simulink model "fft_4096c_1i_core"  (R2019a)
(part 5 of 150)

  butterfly3_7 : Subsystem  AncestorBlock=casper_library_ffts/butterfly_direct  mask(butterfly_direct){n_inputs=1, biplex=off, FFTSize=13, Coeffs=[ 7 2055 1031 3079 519 2567 1543 3591 263 2311 1287 3335 775 2823 1799 3847 135 2183 1159 3207 647 2695 1671 3719 391 2439 1415 3463 903 2951 1927 3975 71 2119 1095 3143 583 2631 1607 3655 327 2375 1351 3399 839 2887 1863 3911 199 2247 1223 3271 711 2759 1735 3783 455 2503 1479 3527 967 3015 1991 4039 39 2087 1063 3111 551 2599 1575 3623 295 2343 1319 3367 807 2855 1831 3879 167 2215 1191 3239 679 2727 1703 3751 423 2471 1447 3495 935 2983 1959 4007 103 2151 1127 3175 615 2663 1639 3687 359 2407 1383 3431 871 2919 1895 3943 231 2279 1255 3303 743 2791 1767 3815 487 2535 1511 3559 999 3047 2023 4071 23 2071 1047 3095 535 2583 1559 3607 279 2327 1303 3351 791 2839 1815 3863 151 2199 1175 3223 663 2711 1687 3735 407 2455 1431 3479 919 2967 1943 3991 87 2135 1111 3159 599 2647 1623 3671 343 2391 1367 3415 855 2903 1879 3927 215 2263 1239 3287 727 2775 1751 3799 471 2519 1495 3543 983 3031 2007 4055 55 2103 1079 3127 567 2615 1591 3639 311 2359 1335 3383 823 2871 1847 3895 183 2231 1207 3255 695 2743 1719 3767 439 2487 1463 3511 951 2999 1975 4023 119 2167 1143 3191 631 2679 1655 3703 375 2423 1399 3447 887 2935 1911 3959 247 2295 1271 3319 759 2807 1783 3831 503 2551 1527 3575 1015 3063 2039 4087 15 2063 1039 3087 527 2575 1551 3599 271 2319 1295 3343 783 2831 1807 3855 143 2191 1167 3215 655 2703 1679 3727 399 2447 1423 3471 911 2959 1935 3983 79 2127 1103 3151 591 2639 1615 3663 335 2383 1359 3407 847 2895 1871 3919 207 2255 1231 3279 719 2767 1743 3791 463 2511 1487 3535 975 3023 1999 4047 47 2095 1071 3119 559 2607 1583 3631 303 2351 1327 3375 815 2863 1839 3887 175 2223 1199 3247 687 2735 1711 3759 431 2479 1455 3503 943 2991 1967 4015 111 2159 1135 3183 623 2671 1647 3695 367 2415 1391 3439 879 2927 1903 3951 239 2287 1263 3311 751 2799 1775 3823 495 2543 1519 3567 1007 3055 2031 4079 31 2079 1055 3103 543 2591 1567 3615 287 2335 1311 3359 799 2847 1823 3871 159 2207 1183 3231 671 2719 1695 3743 415 2463 1439 3487 927 2975 1951 3999 95 2143 1119 3167 607 2655 1631 3679 351 2399 1375 3423 863 2911 1887 3935 223 2271 1247 3295 735 2783 1759 3807 479 2527 1503 3551 991 3039 2015 4063 63 2111 1087 3135 575 2623 1599 3647 319 2367 1343 3391 831 2879 1855 3903 191 2239 1215 3263 703 2751 1727 3775 447 2495 1471 3519 959 3007 1983 4031 127 2175 1151 3199 639 2687 1663 3711 383 2431 1407 3455 895 2943 1919 3967 255 2303 1279 3327 767 2815 1791 3839 511 2559 1535 3583 1023 3071 2047 4095], StepPeriod=0, coeff_bit_width=18, input_bit_width=18, bin_pt_in=17, downshift=off, async=off, floating_point=off, float_type=single, exp_width=8, frac_width=24, add_latency=1, mult_latency=2, bram_latency=2, conv_latency=0, add_pipe_latency=0, mult_pipe_latency=0, quantization=Round  (unbiased: Even Values), overflow=Wrap, coeffs_bit_limit=8, coeff_sharing=on, coeff_decimation=on, coeff_generation=off, cal_bits=1, n_bits_rotation=25, max_fanout=8, use_hdl=on, use_embedded=off, bitgrowth=off, hardcode_shifts=off, dsp48_adders=off}
      mask prompts: n_inputs "number inputs"; biplex "Used in biplex FFT"; FFTSize "Size of FFT: (2^? pts)"; Coeffs "Coefficients: (0 to 2^(FFTSize-1)-1)"; StepPeriod "Coefficient Step Period: (2^?)"; coeff_bit_width "Coefficient Bit Width"; input_bit_width "Input Bit Width"; bin_pt_in "Input binary point"; async "asynchronous operation"; floating_point "floating point"; float_type "float type"; exp_width "exponent width"; frac_width "fraction width"; add_latency "Add Latency"; mult_latency "Mult Latency"; bram_latency "BRAM Latency"; conv_latency "Convert latency"; add_pipe_latency "Add Pipeline Latency"; mult_pipe_latency "Mult Pipeline Latency"; quantization "Quantization Behavior"; overflow "Overflow Behavior"; coeffs_bit_limit "Number bits above which to store stage's coefficients in BRAM (2^? bits)"; coeff_sharing "BRAM sharing in coeff storage"; coeff_decimation "Store a fraction of coeff factors where useful"; coeff_generation "Generate coeffs with multipliers where useful"; cal_bits "Number calibration locations when generating coeffs (2^?)"; n_bits_rotation "Feedback rotation vector resolution"; max_fanout "Maximum fanout"; use_hdl "Use behavioural HDL for multipliers"; use_embedded "Use embedded multipliers"; bitgrowth "Bit growth instead of shifting"; hardcode_shifts "Hardcode shift schedule"; dsp48_adders "Use DSP48s for adders"
      mask help: FFT internal block.
      mask init: same as fft_4096c_1i_core/fft_wideband_real1/fft_direct/butterfly0_0
      settings: AttributesFormatString=twiddle_general
      mask Callback floating_point:
      | onoff = get_param(gcb, 'floating_point');
      | if strcmp(onoff,'on')
      |     enable_fixpt = 'off';
      |     set_param_state(gcb, 'float_type', 'on')
      | 
      |     f_type = get_param(gcb, 'float_type');
      |     if strcmp(f_type,'custom')
      |         set_param_state(gcb, 'exp_width', 'on')
      |         set_param_state(gcb, 'frac_width', 'on')
      |     else
      |         set_param_state(gcb, 'exp_width', 'off')
      |         set_param_state(gcb, 'frac_width', 'off')
      |     end
      | 
      | 
      | else
      |     enable_fixpt = 'on';
      |     set_param_state(gcb, 'float_type', 'off')
      |     set_param_state(gcb, 'exp_width', 'off')
      |     set_param_state(gcb, 'frac_width', 'off')
      | end
      | 
      | set_param_state(gcb, 'input_bit_width', enable_fixpt)
      | set_param_state(gcb, 'bin_pt_in', enable_fixpt)
      | set_param_state(gcb, 'coeff_bit_width', enable_fixpt)
      mask TypeOptions float_type: single | custom
      mask Callback float_type:
      | f_type = get_param(gcb, 'float_type')
      | if strcmp(f_type,'custom')
      |     set_param_state(gcb, 'exp_width', 'on')
      |     set_param_state(gcb, 'frac_width', 'on')
      | else
      |     set_param_state(gcb, 'exp_width', 'off')
      |     set_param_state(gcb, 'frac_width', 'off')
      | end
      mask TypeOptions quantization: Truncate | Round  (unbiased: +/- Inf) | Round  (unbiased: Even Values)
      mask TypeOptions overflow: Wrap | Saturate | Error
      mask Callback use_hdl:
      | % make mutually exclusive with use_embedded.
      | 
      | use_hdl = get_param(gcb, 'use_hdl');
      | if strcmp(use_hdl, 'on'),
      |     set_param_state(gcb, 'use_embedded', 'off');
      | else
      |     set_param_state(gcb, 'use_embedded', 'on');
      | end
      mask Callback use_embedded:
      | % make mutually exclusive with use_hdl.
      | 
      | use_hdl = get_param(gcb, 'use_embedded');
      | if strcmp(use_hdl, 'on'),
      |     set_param_state(gcb, 'use_hdl', 'off');
      | else
      |     set_param_state(gcb, 'use_hdl', 'on');
      | end
      mask Callback hardcode_shifts:
      | hardcode_shifts = get_param(gcb, 'hardcode_shifts');
      | set_param_state(gcb, 'downshift', hardcode_shifts);
      mask Callback dsp48_adders: %fft_callback_dsp48_adders(gcb);
      mask DialogControl ParameterTabVar0 Prompt: Basic
      mask DialogControl ParameterTabVar01 Prompt: Latency
      mask DialogControl ParameterTabVar012 Prompt: Implementation
  combine : xbsIndex_r4/Logical  logical_function=OR  inputs=8  en=off  latency=2  precision=Full  arith_type=Unsigned  n_bits=16  bin_pt=0  align_bp=on  dbl_ovrd=off  block_type=logical
  of_0 : xbsIndex_r4/Delay  rst=off  infoeditControl=Selection of Reset will increase slice count due to use of real FFs and instead of SRLs  en=off  latency=0  reg_retiming=on  dbl_ovrd=off  block_type=delay
  of_1 : xbsIndex_r4/Concat  num_inputs=2  dbl_ovrd=off  block_type=concat
  of_2 : xbsIndex_r4/Concat  num_inputs=4  dbl_ovrd=off  block_type=concat
  of_3 : xbsIndex_r4/Concat  num_inputs=8  dbl_ovrd=off  block_type=concat
  of_expand : Subsystem  AncestorBlock=casper_library_flow_control/bus_expand  mask(bus_expand){mode=divisions of equal size, outputNum=8, outputWidth=1, outputBinaryPt=0, outputArithmeticType=0, show_format=off, outputToWorkspace=off, variablePrefix=out, outputToModelAsWell=on}
      mask prompts: outputNum "Number of outputs:"; outputWidth "Output width:"; outputBinaryPt "Output binary point position:"; outputArithmeticType "Output arithmetic type (ufix=0, fix=1, bool=2):"; show_format "Print format string?"; outputToWorkspace "Output to workspace?"; variablePrefix "Variable name prefix:"; outputToModelAsWell "Output to model as well?"
      mask help:
      | Expands a 'bus' made using a bus_create or Xilinx
      | concat block.
      | The input will be divided into the specified number
      | of outputs with the specified arithmetic types.
      | Divisions are made from most significant bit.
      mask init: same as fft_4096c_1i_core/bus_expand
      settings: AttributesFormatString=8 outputs
      mask TypeOptions mode: divisions of equal size | divisions of arbitrary size
      mask Callback mode: bus_expand_callback();
      mask Callback outputWidth: bus_expand_callback();
      mask Callback outputToWorkspace: bus_expand_callback();
  of_or : xbsIndex_r4/Logical  logical_function=OR  inputs=4  en=off  latency=2  precision=Full  arith_type=Unsigned  n_bits=16  bin_pt=0  align_bp=on  dbl_ovrd=off  block_type=logical
  slice0 : xbsIndex_r4/Slice  nbits=1  boolean_output=on  mode=Lower Bit Location + Width  bit1=0  base1=MSB of Input  bit0=0  base0=LSB of Input  dbl_ovrd=off  block_type=slice
  slice1 : xbsIndex_r4/Slice  nbits=1  boolean_output=on  mode=Lower Bit Location + Width  bit1=0  base1=MSB of Input  bit0=1  base0=LSB of Input  dbl_ovrd=off  block_type=slice
  slice2 : xbsIndex_r4/Slice  nbits=1  boolean_output=on  mode=Lower Bit Location + Width  bit1=0  base1=MSB of Input  bit0=2  base0=LSB of Input  dbl_ovrd=off  block_type=slice
  slice3 : xbsIndex_r4/Slice  nbits=1  boolean_output=on  mode=Lower Bit Location + Width  bit1=0  base1=MSB of Input  bit0=3  base0=LSB of Input  dbl_ovrd=off  block_type=slice
  synct{1..7} (7 alike) : Terminator
  sync_out : Outport
  out00 : Outport  Port=2
  out01 : Outport  Port=3
  out02 : Outport  Port=4
  out03 : Outport  Port=5
  out04 : Outport  Port=6
  out05 : Outport  Port=7
  out06 : Outport  Port=8
  out07 : Outport  Port=9
  out08 : Outport  Port=10
  out09 : Outport  Port=11
  out010 : Outport  Port=12
  out011 : Outport  Port=13
  out012 : Outport  Port=14
  out013 : Outport  Port=15
  out014 : Outport  Port=16
  out015 : Outport  Port=17
  of : Outport  Port=18
  wires:
  in00/1 -> abus/1(in1)
  adebus3_0/1(msb_lsb_out1) -> out00/1
  in01/1 -> abus/2(in2)
  adebus3_4/1(msb_lsb_out1) -> out01/1
  in02/1 -> abus/3(in3)
  adebus3_2/1(msb_lsb_out1) -> out02/1
  in03/1 -> abus/4(in4)
  adebus3_6/1(msb_lsb_out1) -> out03/1
  in04/1 -> abus/5(in5)
  adebus3_1/1(msb_lsb_out1) -> out04/1
  in05/1 -> abus/6(in6)
  adebus3_5/1(msb_lsb_out1) -> out05/1
  in06/1 -> abus/7(in7)
  adebus3_3/1(msb_lsb_out1) -> out06/1
  in07/1 -> abus/8(in8)
  adebus3_7/1(msb_lsb_out1) -> out07/1
  in08/1 -> bbus/1(in1)
  bdebus3_0/1(msb_lsb_out1) -> out08/1
  in09/1 -> bbus/2(in2)
  bdebus3_4/1(msb_lsb_out1) -> out09/1
  in010/1 -> bbus/3(in3)
  bdebus3_2/1(msb_lsb_out1) -> out010/1
  in011/1 -> bbus/4(in4)
  bdebus3_6/1(msb_lsb_out1) -> out011/1
  in012/1 -> bbus/5(in5)
  bdebus3_1/1(msb_lsb_out1) -> out012/1
  in013/1 -> bbus/6(in6)
  bdebus3_5/1(msb_lsb_out1) -> out013/1
  in014/1 -> bbus/7(in7)
  bdebus3_3/1(msb_lsb_out1) -> out014/1
  in015/1 -> bbus/8(in8)
  bdebus3_7/1(msb_lsb_out1) -> out015/1
  of_or/1 -> of_expand/1(bus_in)
  of_expand/1(msb_out8) -> combine/1
  of_expand/2(out7) -> combine/2
  of_expand/3(out6) -> combine/3
  of_expand/4(out5) -> combine/4
  of_expand/5(out4) -> combine/5
  of_expand/6(out3) -> combine/6
  of_expand/7(out2) -> combine/7
  of_expand/8(lsb_out1) -> combine/8
  combine/1 -> of/1
  shift/1 -> slice0/1, slice1/1, slice2/1, slice3/1
  of_0/1 -> of_or/1
  sync/1 -> butterfly0_0/3(sync_in)
  slice0/1 -> butterfly0_0/4(shift)
  abus/1(bus_out) -> butterfly0_0/1(a)
  bbus/1(bus_out) -> butterfly0_0/2(b)
  butterfly0_0/3(of) -> of_0/1
  butterfly0_0/1(a+bw) -> adebus0_0/1(bus_in)
  butterfly0_0/2(a-bw) -> bdebus0_0/1(bus_in)
  of_1/1 -> of_or/2
  butterfly0_0/4(sync_out) -> butterfly1_0/3(sync_in), butterfly1_1/3(sync_in)
  slice1/1 -> butterfly1_0/4(shift), butterfly1_1/4(shift)
  adebus0_0/1(msb_out2) -> butterfly1_0/1(a)
  adebus0_0/2(lsb_out1) -> butterfly1_0/2(b)
  butterfly1_0/3(of) -> of_1/1
  butterfly1_0/1(a+bw) -> adebus1_0/1(bus_in)
  butterfly1_0/2(a-bw) -> bdebus1_0/1(bus_in)
  bdebus0_0/1(msb_out2) -> butterfly1_1/1(a)
  bdebus0_0/2(lsb_out1) -> butterfly1_1/2(b)
  butterfly1_1/3(of) -> of_1/2
  butterfly1_1/1(a+bw) -> adebus1_1/1(bus_in)
  butterfly1_1/2(a-bw) -> bdebus1_1/1(bus_in)
  of_2/1 -> of_or/3
  butterfly1_0/4(sync_out) -> butterfly2_0/3(sync_in), butterfly2_1/3(sync_in)
  slice2/1 -> butterfly2_0/4(shift), butterfly2_1/4(shift), butterfly2_2/4(shift), butterfly2_3/4(shift)
  adebus1_0/1(msb_out2) -> butterfly2_0/1(a)
  adebus1_0/2(lsb_out1) -> butterfly2_0/2(b)
  butterfly2_0/3(of) -> of_2/1
  butterfly2_0/1(a+bw) -> adebus2_0/1(bus_in)
  butterfly2_0/2(a-bw) -> bdebus2_0/1(bus_in)
  bdebus1_0/1(msb_out2) -> butterfly2_1/1(a)
  bdebus1_0/2(lsb_out1) -> butterfly2_1/2(b)
  butterfly2_1/3(of) -> of_2/2
  butterfly2_1/1(a+bw) -> adebus2_1/1(bus_in)
  butterfly2_1/2(a-bw) -> bdebus2_1/1(bus_in)
  butterfly1_1/4(sync_out) -> butterfly2_2/3(sync_in), butterfly2_3/3(sync_in)
  adebus1_1/1(msb_out2) -> butterfly2_2/1(a)
  adebus1_1/2(lsb_out1) -> butterfly2_2/2(b)
  butterfly2_2/3(of) -> of_2/3
  butterfly2_2/1(a+bw) -> adebus2_2/1(bus_in)
  butterfly2_2/2(a-bw) -> bdebus2_2/1(bus_in)
  bdebus1_1/1(msb_out2) -> butterfly2_3/1(a)
  bdebus1_1/2(lsb_out1) -> butterfly2_3/2(b)
  butterfly2_3/3(of) -> of_2/4
  butterfly2_3/1(a+bw) -> adebus2_3/1(bus_in)
  butterfly2_3/2(a-bw) -> bdebus2_3/1(bus_in)
  of_3/1 -> of_or/4
  butterfly2_0/4(sync_out) -> butterfly3_0/3(sync_in), butterfly3_1/3(sync_in)
  butterfly3_0/4(sync_out) -> sync_out/1
  slice3/1 -> butterfly3_0/4(shift), butterfly3_1/4(shift), butterfly3_2/4(shift), butterfly3_3/4(shift), butterfly3_4/4(shift), butterfly3_5/4(shift), butterfly3_6/4(shift), butterfly3_7/4(shift)
  adebus2_0/1(msb_out2) -> butterfly3_0/1(a)
  adebus2_0/2(lsb_out1) -> butterfly3_0/2(b)
  butterfly3_0/3(of) -> of_3/1
  butterfly3_1/4(sync_out) -> synct1/1
  bdebus2_0/1(msb_out2) -> butterfly3_1/1(a)
  bdebus2_0/2(lsb_out1) -> butterfly3_1/2(b)
  butterfly3_1/3(of) -> of_3/2
  butterfly2_1/4(sync_out) -> butterfly3_2/3(sync_in), butterfly3_3/3(sync_in)
  butterfly3_2/4(sync_out) -> synct2/1
  adebus2_1/1(msb_out2) -> butterfly3_2/1(a)
  adebus2_1/2(lsb_out1) -> butterfly3_2/2(b)
  butterfly3_2/3(of) -> of_3/3
  butterfly3_3/4(sync_out) -> synct3/1
  bdebus2_1/1(msb_out2) -> butterfly3_3/1(a)
  bdebus2_1/2(lsb_out1) -> butterfly3_3/2(b)
  butterfly3_3/3(of) -> of_3/4
  butterfly2_2/4(sync_out) -> butterfly3_4/3(sync_in), butterfly3_5/3(sync_in)
  butterfly3_4/4(sync_out) -> synct4/1
  adebus2_2/1(msb_out2) -> butterfly3_4/1(a)
  adebus2_2/2(lsb_out1) -> butterfly3_4/2(b)
  butterfly3_4/3(of) -> of_3/5
  butterfly3_5/4(sync_out) -> synct5/1
  bdebus2_2/1(msb_out2) -> butterfly3_5/1(a)
  bdebus2_2/2(lsb_out1) -> butterfly3_5/2(b)
  butterfly3_5/3(of) -> of_3/6
  butterfly2_3/4(sync_out) -> butterfly3_6/3(sync_in), butterfly3_7/3(sync_in)
  butterfly3_6/4(sync_out) -> synct6/1
  adebus2_3/1(msb_out2) -> butterfly3_6/1(a)
  adebus2_3/2(lsb_out1) -> butterfly3_6/2(b)
  butterfly3_6/3(of) -> of_3/7
  butterfly3_7/4(sync_out) -> synct7/1
  bdebus2_3/1(msb_out2) -> butterfly3_7/1(a)
  bdebus2_3/2(lsb_out1) -> butterfly3_7/2(b)
  butterfly3_7/3(of) -> of_3/8
  butterfly3_0/1(a+bw) -> adebus3_0/1(bus_in)
  butterfly3_0/2(a-bw) -> bdebus3_0/1(bus_in)
  butterfly3_1/1(a+bw) -> adebus3_1/1(bus_in)
  butterfly3_1/2(a-bw) -> bdebus3_1/1(bus_in)
  butterfly3_2/1(a+bw) -> adebus3_2/1(bus_in)
  butterfly3_2/2(a-bw) -> bdebus3_2/1(bus_in)
  butterfly3_3/1(a+bw) -> adebus3_3/1(bus_in)
  butterfly3_3/2(a-bw) -> bdebus3_3/1(bus_in)
  butterfly3_4/1(a+bw) -> adebus3_4/1(bus_in)
  butterfly3_4/2(a-bw) -> bdebus3_4/1(bus_in)
  butterfly3_5/1(a+bw) -> adebus3_5/1(bus_in)
  butterfly3_5/2(a-bw) -> bdebus3_5/1(bus_in)
  butterfly3_6/1(a+bw) -> adebus3_6/1(bus_in)
  butterfly3_6/2(a-bw) -> bdebus3_6/1(bus_in)
  butterfly3_7/1(a+bw) -> adebus3_7/1(bus_in)
  butterfly3_7/2(a-bw) -> bdebus3_7/1(bus_in)
